simulink model "generic_truck"  (R2025a)
settings: Solver=VariableStepAuto  StartTime=0.0  StopTime=600  FixedStep=0.01  MaxStep=0.001  RelTol=1e-3  EnableMultiTasking=on
libraries: TruckMaker4SL x205, simulink x1
(part 6 of 9)

== matlab function generic_truck/TruckMaker/Two_TRack_Model/Two Track Model ==
  data: z input; u input; Q input; R input; xhat output; Ts input; P_out output; Fy_mean output; alpha_mean output; V_FL_whl output; V_FR_whl output; V_RL_whl output; V_RR_whl output
function [xhat,P_out,Fy_mean,alpha_mean,...
          V_FL_whl,V_FR_whl,V_RL_whl,V_RR_whl] ...
          = UKF_4Wheel(z,u,Q,R,Ts)

persistent x P

%% ================= INIT =================
if isempty(x)
    x = [15; 0; 0.01; 4; 4; 4; 4];
end

if isempty(P)
    P = diag([1 1 0.01 1e4 1e4 1e4 1e4]);
end

n = length(x);
m = length(z);

%% ================= VEHICLE =================
m_car = 7000;
Jz = 14232.357;
lf = 4.52;
lr = 0.95;
R_w = 0.49;
track=2.10;

%% ================= INPUTS =================
delta_FL = u(1);
delta_FR = u(2);
delta_RL = 0;
delta_RR = 0;

Fx_FL = u(5)/R_w;
Fx_FR = u(6)/R_w;
Fx_RL = u(7)/R_w;
Fx_RR = u(8)/R_w;

%% ================= ROTATION MATRICES =================
R_FL = [cos(delta_FL) sin(delta_FL);
       -sin(delta_FL) cos(delta_FL)];

R_FR = [cos(delta_FR) sin(delta_FR);
       -sin(delta_FR) cos(delta_FR)];

R_RL = eye(2);
R_RR = eye(2);

%% ================= GEOMETRY =================
tire_FL = [lf;  1.05; 0];
tire_FR = [lf; -1.05; 0];
tire_RL = [lr;  1.05; 0];
tire_RR = [lr; -1.05; 0];

CoM = [3.6; 0; 1];  % Ändra koor till COM (Jobba i CoG)  

rFL = tire_FL - CoM;
rFR = tire_FR - CoM;
rRL = tire_RL - CoM;
rRR = tire_RR - CoM;

%% ================= UKF =================
W0 = 1 - n/3;
Wi = (1 - W0)/(2*n);
gamma = sqrt(n/(1-W0));

%P = (P+P')/2 + 1e-9*eye(n); 
S = chol(P,'lower'); %% kolla upp den igen 

X = zeros(n,2*n+1);
X(:,1) = x;

for i=1:n
    X(:,i+1)   = x + gamma*S(:,i);
    X(:,i+1+n) = x - gamma*S(:,i);
end

%% ================= PROPAGATION =================
X_pred = zeros(n,2*n+1);
Fy_sigma = zeros(4,2*n+1);
alpha_sigma = zeros(4,2*n+1);
% R; M; Jz
for k=1:2*n+1

    vx = X(1,k);
    vy = X(2,k);
    r  = X(3,k);

    Cf_FL = X(4,k);
    Cf_FR = X(5,k);
    Cr_RL = X(6,k);
    Cr_RR = X(7,k);

    % ===== FIX 1: korrekt vx_safe =====
    %vx_safe = vx;

    Vc = [vx; vy; 0]; % vehilce Frame 
    omega = [0;0;r];

    V_FL = Vc + cross(omega,rFL);
    V_FR = Vc + cross(omega,rFR);
    V_RL = Vc + cross(omega,rRL);
    V_RR = Vc + cross(omega,rRR);

    V_FL_l = R_FL*V_FL(1:2);
    V_FR_l = R_FR*V_FR(1:2);
    V_RL_l = V_RL(1:2);
    V_RR_l = V_RR(1:2);
    
    %============Side Slip Vinkel på respektiv däck ==================
    alpha_FL = atan2(V_FL_l(2),max(abs(V_FL_l(1)),0.1));
    alpha_FR = atan2(V_FR_l(2),max(abs(V_FR_l(1)),0.1));
    alpha_RL = atan2(V_RL_l(2),max(abs(V_RL_l(1)),0.1));
    alpha_RR = atan2(V_RR_l(2),max(abs(V_RR_l(1)),0.1));


    %===================Forces==============================
    Fy_FL = -Cf_FL*alpha_FL;
    Fy_FR = -Cf_FR*alpha_FR;
    Fy_RL = -Cr_RL*alpha_RL;
    Fy_RR = -Cr_RR*alpha_RR;


    % Transformerta dessa krafter till kroppens FRAME
    F_FL = R_FL'*[Fx_FL;Fy_FL];
    F_FR = R_FR'*[Fx_FR;Fy_FR];
    F_RL = [Fx_RL;Fy_RL];
    F_RR = [Fx_RR;Fy_RR];

    Fx_sum = F_FL(1)+F_FR(1)+F_RL(1)+F_RR(1);
    Fy_sum = F_FL(2)+F_FR(2)+F_RL(2)+F_RR(2);

    dvx = Fx_sum/m_car + vy*r; % andra terma roteradnde koordinat system 
    dvy = Fy_sum/m_car - vx*r; 

%dW = truck.Jinv * (cross(R1, RotW1*F1) + cross(R2, RotW2*F2) 
                    % + cross(R3, F3) + cross(R4, F4));

    % ===== FIX 2: korrekt  eller ej fråga Axel  yaw moment =====
    % !!!!!!!!!!
    Mz = (lf-CoM(1))*(F_FL(2)+F_FR(2)) - (CoM(1)-lr)*(F_RL(2)+F_RR(2)) ... 
        + (track/2)*(F_FR(1)-F_FL(1)) + (track/2)*(F_RR(1)-F_RL(1));
    dr = Mz / Jz;

    X_pred(:,k) = [vx+dvx*Ts;
                   vy+dvy*Ts;
                   r+dr*Ts;
                   Cf_FL;
                   Cf_FR;
                   Cr_RL;
                   Cr_RR];

    Fy_sigma(:,k)    = [F_FL(2);F_FR(2);F_RL(2);F_RR(2)];
    alpha_sigma(:,k) = [alpha_FL;alpha_FR;alpha_RL;alpha_RR];
end

W = [W0 repmat(Wi,1,2*n)];
%x_pred = X_pred*W';
Fy_mean = Fy_sigma*W';
alpha_mean = alpha_sigma*W';
%% Predicted mean
x_pred = W0*X_pred(:,1);
for k=2:2*n+1
    x_pred = x_pred + Wi*X_pred(:,k);
end

%% ================= COVARIANCE =================
% P_pred = Q*Ts;
% for k=1:2*n+1
%     dx = X_pred(:,k)-x_pred;
%     P_pred = P_pred + W(k)*(dx*dx');
% end

%% Predicted covariance
P_pred = Q*Ts;
for k=1:2*n+1
    w = (k==1)*W0 + (k>1)*Wi;
    dx = X_pred(:,k) - x_pred;
    P_pred = P_pred + w*(dx*dx');
end
%% ================= MEASUREMENT =================
Z_sigma = zeros(m,2*n+1);

for k=1:2*n+1

    vx = X_pred(1,k);
    vy = X_pred(2,k);
    r  = X_pred(3,k);

    %Cf_FL = X_pred(4,k);
    %Cf_FR = X_pred(5,k);
    %Cr_RL = X_pred(6,k);
    %Cr_RR = X_pred(7,k);


    vx_safe = abs(vx);

    Vc = [vx_safe;vy;0];
    omega = [0;0;r];

    V_FL = Vc + cross(omega,rFL);
    V_FR = Vc + cross(omega,rFR);
    V_RL = Vc + cross(omega,rRL);
    V_RR = Vc + cross(omega,rRR);

    V_FL_l = R_FL*V_FL(1:2);
    V_FR_l = R_FR*V_FR(1:2);
    V_RL_l = V_RL(1:2);
    V_RR_l = V_RR(1:2);

     %============Side Slip Vinkel på respektiv däck ==================
    alpha_FL = atan2(V_FL_l(2),max(abs(V_FL_l(1)),0.1));
    alpha_FR = atan2(V_FR_l(2),max(abs(V_FR_l(1)),0.1));
    alpha_RL = atan2(V_RL_l(2),max(abs(V_RL_l(1)),0.1));
    alpha_RR = atan2(V_RR_l(2),max(abs(V_RR_l(1)),0.1));


    %===================Forces==============================
    Fy_FL = -Cf_FL*alpha_FL;
    Fy_FR = -Cf_FR*alpha_FR;
    Fy_RL = -Cr_RL*alpha_RL;
    Fy_RR = -Cr_RR*alpha_RR;


    % Transformerta dessa krafter till kroppens FRAME
    F_FL = R_FL'*[Fx_FL;Fy_FL];
    F_FR = R_FR'*[Fx_FR;Fy_FR];
    F_RL = [Fx_RL;Fy_RL];
    F_RR = [Fx_RR;Fy_RR];

    Fx_sum = F_FL(1)+F_FR(1)+F_RL(1)+F_RR(1);
    Fy_sum = F_FL(2)+F_FR(2)+F_RL(2)+F_RR(2);

    % ===== FIX 3: hjulhastigheter istället för krafter =====
    w_FL = V_FL_l(1)/R_w;    % Fråga MATS om Long slip och R_w 
    w_FR = V_FR_l(1)/R_w;
    w_RL = V_RL_l(1)/R_w;
    w_RR = V_RR_l(1)/R_w;

    ax = (Fx_sum)/m_car ;
    ay = (Fy_sum)/m_car;

    Z_sigma(:,k) = [ax; ay; vx; vy; r; w_FL; w_FR; w_RL; w_RR];
end

% z_pred = Z_sigma*W';
% 
% P_zz = R;
% P_xz = zeros(n,m);
% 
% for k=1:2*n+1
%     dz = Z_sigma(:,k)-z_pred;
%     dx = X_pred(:,k)-x_pred;
%     P_zz = P_zz + W(k)*(dz*dz');
%     P_xz = P_xz + W(k)*(dx*dz');
% end
% 
% %% ================= UPDATE =================
% K =   P_xz / P_zz;
% x = x_pred + K*(z - z_pred);
% 
% P = P_pred - K*P_zz*K';

% ===== FIX 4: symmetrisera P =====
%P = (P+P')/2 + 1e-9*eye(n);

%% Measurement mean
z_pred = W0*Z_sigma(:,1);
for k=2:2*n+1
    z_pred = z_pred + Wi*Z_sigma(:,k);
end

%% Measurement covariance
S_cov = R;
for k=1:2*n+1
    w = (k==1)*W0 + (k>1)*Wi;
    dz = Z_sigma(:,k) - z_pred;
    S_cov = S_cov + w*(dz*dz');
end

%% Cross covariance
Pxz = zeros(n,length(z));
for k=1:2*n+1
    w = (k==1)*W0 + (k>1)*Wi;
    dx = X_pred(:,k) - x_pred;
    dz = Z_sigma(:,k) - z_pred;
    Pxz = Pxz + w*(dx*dz');
end

%% Kalman update
K = Pxz / (S_cov);
x = x_pred + K*(z - z_pred);
P = P_pred - K*S_cov*K';

%% ================= OUTPUT =================
vx = x(1); vy = x(2); r = x(3);

Vc = [vx;vy;0];
omega = [0;0;r];

V_FL = Vc + cross(omega,rFL);
V_FR = Vc + cross(omega,rFR);
V_RL = Vc + cross(omega,rRL);
V_RR = Vc + cross(omega,rRR);

V_FL_whl = R_FL*V_FL(1:2);
V_FR_whl = R_FR*V_FR(1:2);
V_RL_whl = V_RL(1:2);
V_RR_whl = V_RR(1:2);

xhat =  x;
P_out = P;

end

== matlab function generic_truck/TruckMaker/Two_TRack_Model/Two Track Model1 ==
  data: z input; u input; Q input; R input; xhat output; Ts input; P_out output; Fy_mean output; alpha_mean output; V_FL_whl output; V_FR_whl output; V_RL_whl output; V_RR_whl output
function [xhat,P_out,Fy_mean,alpha_mean,...
          V_FL_whl,V_FR_whl,V_RL_whl,V_RR_whl] ...
          = UKF_4Wheel(z,u,Q,R,Ts)

persistent x P

%% ================= INIT =================
if isempty(x)
    x = [15; 0; 0.01; 10; 10; 10; 10];  % startvärden på cornering stiffness
end

if isempty(P)
    P = diag([1 1 0.01 1 1 1 1]);
end

n = length(x);
m = length(z);

%% ================= VEHICLE =================
m_car = 7000;
Jz = 14232.357;
lf = 4.52;
lr = 0.95;
R_w = 0.49;
track=2.10;
h_CoM = 1;  % höjd på CoM

%% ================= INPUTS =================
delta_FL = u(1);
delta_FR = u(2);
delta_RL = 0;
delta_RR = 0;

Fx_FL = u(5)/R_w;
Fx_FR = u(6)/R_w;
Fx_RL = u(7)/R_w;
Fx_RR = u(8)/R_w;

%% ================= ROTATION MATRICES =================
R_FL = [cos(delta_FL) sin(delta_FL);
       -sin(delta_FL) cos(delta_FL)];

R_FR = [cos(delta_FR) sin(delta_FR);
       -sin(delta_FR) cos(delta_FR)];

R_RL = eye(2);
R_RR = eye(2);

%% ================= GEOMETRY =================
tire_FL = [lf;  track/2; 0];
tire_FR = [lf; -track/2; 0];
tire_RL = [lr;  track/2; 0];
tire_RR = [lr; -track/2; 0];

CoM = [3.6; 0; h_CoM];  

rFL = tire_FL - CoM;
rFR = tire_FR - CoM;
rRL = tire_RL - CoM;
rRR = tire_RR - CoM;

%% ================= UKF =================
W0 = 1 - n/3;
Wi = (1 - W0)/(2*n);
gamma = sqrt(n/(1-W0));

S = chol(P,'lower');

X = zeros(n,2*n+1);
X(:,1) = x;

for i=1:n
    X(:,i+1)   = x + gamma*S(:,i);
    X(:,i+1+n) = x - gamma*S(:,i);
end

%% ================= PROPAGATION =================
X_pred = zeros(n,2*n+1);
Fy_sigma = zeros(4,2*n+1);
alpha_sigma = zeros(4,2*n+1);

for k=1:2*n+1

    vx = X(1,k);
    vy = X(2,k);
    r  = X(3,k);

    Cf_FL = X(4,k);
    Cf_FR = X(5,k);
    Cr_RL = X(6,k);
    Cr_RR = X(7,k);

    Vc = [vx; vy; 0];
    omega = [0;0;r];

    V_FL = Vc + cross(omega,rFL);
    V_FR = Vc + cross(omega,rFR);
    V_RL = Vc + cross(omega,rRL);
    V_RR = Vc + cross(omega,rRR);

    V_FL_l = R_FL*V_FL(1:2);
    V_FR_l = R_FR*V_FR(1:2);
    V_RL_l = V_RL(1:2);
    V_RR_l = V_RR(1:2);
    
    % Side slip angles
    alpha_FL = atan2(V_FL_l(2),max(abs(V_FL_l(1)),0.1));
    alpha_FR = atan2(V_FR_l(2),max(abs(V_FR_l(1)),0.1));
    alpha_RL = atan2(V_RL_l(2),max(abs(V_RL_l(1)),0.1));
    alpha_RR = atan2(V_RR_l(2),max(abs(V_RR_l(1)),0.1));

    % ================= LOAD TRANSFER =================
    Fz_FL = m_car/4*9.81 - m_car*r*vy - m_car*vx^2*lr/(lf+lr); % enkel approx
    Fz_FR = m_car/4*9.81 - m_car*r*vy - m_car*vx^2*lr/(lf+lr);
    Fz_RL = m_car/4*9.81 + m_car*r*vy + m_car*vx^2*lf/(lf+lr);
    Fz_RR = m_car/4*9.81 + m_car*r*vy + m_car*vx^2*lf/(lf+lr);

    % ================= FORCES =================
    Fy_FL = -Cf_FL * Fz_FL * alpha_FL;
    Fy_FR = -Cf_FR * Fz_FR * alpha_FR;
    Fy_RL = -Cr_RL * Fz_RL * alpha_RL;
    Fy_RR = -Cr_RR * Fz_RR * alpha_RR;

    F_FL = R_FL'*[Fx_FL;Fy_FL];
    F_FR = R_FR'*[Fx_FR;Fy_FR];
    F_RL = [Fx_RL;Fy_RL];
    F_RR = [Fx_RR;Fy_RR];

    Fx_sum = F_FL(1)+F_FR(1)+F_RL(1)+F_RR(1);
    Fy_sum = F_FL(2)+F_FR(2)+F_RL(2)+F_RR(2);

    dvx = Fx_sum/m_car + vy*r;
    dvy = Fy_sum/m_car - vx*r;

    Mz = (lf-CoM(1))*(F_FL(2)+F_FR(2)) - (CoM(1)-lr)*(F_RL(2)+F_RR(2)) ...
        + (track/2)*(F_FR(1)-F_FL(1)) + (track/2)*(F_RR(1)-F_RL(1));
    dr = Mz / Jz;

    X_pred(:,k) = [vx+dvx*Ts;
                   vy+dvy*Ts;
                   r+dr*Ts;
                   Cf_FL;
                   Cf_FR;
                   Cr_RL;
                   Cr_RR];

    Fy_sigma(:,k)    = [F_FL(2);F_FR(2);F_RL(2);F_RR(2)];
    alpha_sigma(:,k) = [alpha_FL;alpha_FR;alpha_RL;alpha_RR];
end

%% ================= UKF MEAN & COVARIANCE =================
W = [W0 repmat(Wi,1,2*n)];
Fy_mean = Fy_sigma*W';
alpha_mean = alpha_sigma*W';

% State mean
x_pred = W0*X_pred(:,1);
for k=2:2*n+1
    x_pred = x_pred + Wi*X_pred(:,k);
end

% State covariance
P_pred = Q*Ts;
for k=1:2*n+1
    w = (k==1)*W0 + (k>1)*Wi;
    dx = X_pred(:,k) - x_pred;
    P_pred = P_pred + w*(dx*dx');
end

%% ================= MEASUREMENT =================
Z_sigma = zeros(m,2*n+1);

for k=1:2*n+1
    vx = X_pred(1,k);
    vy = X_pred(2,k);
    r  = X_pred(3,k);

    Cf_FL = X_pred(4,k);
    Cf_FR = X_pred(5,k);
    Cr_RL = X_pred(6,k);
    Cr_RR = X_pred(7,k);

    Vc = [vx;vy;0];
    omega = [0;0;r];

    V_FL = Vc + cross(omega,rFL);
    V_FR = Vc + cross(omega,rFR);
    V_RL = Vc + cross(omega,rRL);
    V_RR = Vc + cross(omega,rRR);

    V_FL_l = R_FL*V_FL(1:2);
    V_FR_l = R_FR*V_FR(1:2);
    V_RL_l = V_RL(1:2);
    V_RR_l = V_RR(1:2);

    alpha_FL = atan2(V_FL_l(2),max(abs(V_FL_l(1)),0.1));
    alpha_FR = atan2(V_FR_l(2),max(abs(V_FR_l(1)),0.1));
    alpha_RL = atan2(V_RL_l(2),max(abs(V_RL_l(1)),0.1));
    alpha_RR = atan2(V_RR_l(2),max(abs(V_RR_l(1)),0.1));

     % ================= LOAD TRANSFER =================
    Fz_FL = m_car/4*9.81 - m_car*r*vy - m_car*vx^2*lr/(lf+lr); % enkel approx
    Fz_FR = m_car/4*9.81 - m_car*r*vy - m_car*vx^2*lr/(lf+lr);
    Fz_RL = m_car/4*9.81 + m_car*r*vy + m_car*vx^2*lf/(lf+lr);
    Fz_RR = m_car/4*9.81 + m_car*r*vy + m_car*vx^2*lf/(lf+lr);

    Fy_FL = -Cf_FL * Fz_FL * alpha_FL;
    Fy_FR = -Cf_FR * Fz_FR * alpha_FR;
    Fy_RL = -Cr_RL * Fz_RL * alpha_RL;
    Fy_RR = -Cr_RR * Fz_RR * alpha_RR;

    F_FL = R_FL'*[Fx_FL;Fy_FL];
    F_FR = R_FR'*[Fx_FR;Fy_FR];
    F_RL = [Fx_RL;Fy_RL];
    F_RR = [Fx_RR;Fy_RR];

    Fx_sum = F_FL(1)+F_FR(1)+F_RL(1)+F_RR(1);
    Fy_sum = F_FL(2)+F_FR(2)+F_RL(2)+F_RR(2);

    w_FL = V_FL_l(1)/R_w;
    w_FR = V_FR_l(1)/R_w;
    w_RL = V_RL_l(1)/R_w;
    w_RR = V_RR_l(1)/R_w;

    ax = Fx_sum/m_car;
    ay = Fy_sum/m_car;

    Z_sigma(:,k) = [ax; ay; vx; vy; r; w_FL; w_FR; w_RL; w_RR];
end

%% ================= UKF UPDATE =================
% Measurement mean
z_pred = W0*Z_sigma(:,1);
for k=2:2*n+1
    z_pred = z_pred + Wi*Z_sigma(:,k);
end

% Measurement covariance
S_cov = R;
for k=1:2*n+1
    w = (k==1)*W0 + (k>1)*Wi;
    dz = Z_sigma(:,k) - z_pred;
    S_cov = S_cov + w*(dz*dz');
end

% Cross covariance
Pxz = zeros(n,length(z));
for k=1:2*n+1
    w = (k==1)*W0 + (k>1)*Wi;
    dx = X_pred(:,k) - x_pred;
    dz = Z_sigma(:,k) - z_pred;
    Pxz = Pxz + w*(dx*dz');
end

% Kalman update
K = Pxz / S_cov;
x = x_pred + K*(z - z_pred);
P = P_pred - K*S_cov*K';

%% ================= OUTPUT =================
vx = x(1); vy = x(2); r = x(3);

Vc = [vx;vy;0];
omega = [0;0;r];

V_FL = Vc + cross(omega,rFL);
V_FR = Vc + cross(omega,rFR);
V_RL = Vc + cross(omega,rRL);
V_RR = Vc + cross(omega,rRR);

V_FL_whl = R_FL*V_FL(1:2);
V_FR_whl = R_FR*V_FR(1:2);
V_RL_whl = V_RL(1:2);
V_RR_whl = V_RR(1:2);

xhat =  x;
P_out = P;
Fy_mean = Fy_mean;
alpha_mean = alpha_mean;

end

== matlab function generic_truck/TruckMaker/Subsystem1/ONE_TRACK_MODEL_TRACTOR_UKF/MATLAB Function ==
  data: z input; u input; Cf output; Cr output; alpha_f output; alpha_r output
function [Cf, Cr, alpha_f, alpha_r] = stiffness_computation(z, u)
%
% Signal: z = [ ax; ay; az; 
%               vx; vy; vz;
%               rx; ry; rz;
%               alphax; alphay; alphaz;
%               wFL; wFR; wRL; wRR; ]
%
%         u = [ delta; T_rl; T_rr; ]
%

% ------------------------------------------------------------------------%
% Physics
% ------------------------------------------------------------------------%

g = 9.82; % [m/s^2]

% ------------------------------------------------------------------------%
% Truck Parameters
% ------------------------------------------------------------------------%

% Mass [kg]
m = 6800;

% Inertial tensor [kg m^2]
J = [
     5430.025, 0.000,    -589.488;
     0.000,    9407.562,  0.000;
    -589.488,  0.000,     12994.917;
];

% Position vectors [m]
p_cog  = [3.473, 0.000, 0.925].';  % Center of Gravity
p_fax  = [4.520, 0.000, 0.490].';  % Front axle
p_rax  = [0.950, 0.000, 0.490].';  % Rear axle
p_bod  = [3.600, 0.000, 1.000].';  % Body frame
p_imu  = p_bod;

% p_wfl  = [4.520,  1.050, 0.490].'; % Front wheel left
% p_wfr  = [4.520, -1.050, 0.490].'; % Front wheel right
% 
% p_wrl  = [0.950,  1.050, 0.490].'; % Rear wheel left
% p_wrcl = [0.950,  0.860, 0.490].'; % Rear wheel carrier left
% p_wrcr = [0.950, -0.860, 0.490].'; % Rear wheel carrier right
% p_wrr  = [0.950, -1.050, 0.490].'; % Rear wheel right
% 
% Axle load
% m_f = 4805.882; % [kg]
% m_r = 2194.118; % [kg]
% 
% Wheel base
% long = [1,0,0] * abs(p_fax - p_rax); % length [m]
% wide = [0,1,0] * abs(p_wrr - p_wrl); % width  [m]

% CoG hight
high = p_cog(3);

% Wheel radius
% Rwf = 0.505;
% Rwr = 0.505;

% longitudinal distance from cog to axles
lf = [1,0,0] * abs(p_fax - p_cog);
lr = [1,0,0] * abs(p_rax - p_cog);

% ------------------------------------------------------------------------%
% Inputs
% ------------------------------------------------------------------------%

a =  [z(1:2);0]; % IMU acceleration
v =  [z(3:4);0]; % IMU velocity

alpha = [0;0;0];     % IMU yaw acceleration

omega = [0;0;z(end)];  % IMU yaw rate


delta = u(1); % steering angle of one-track front wheel (pre-computed)

T_rl = u(2); % rear left  torque (not used)
T_rr = u(3); % rear right torque (not used)
 
% ------------------------------------------------------------------------%
% Translate measurements
% ------------------------------------------------------------------------%

% displacement vectors
Rfax = p_fax - p_imu; Rfax(3) = -p_imu(3); % straight projection to contact
Rrax = p_rax - p_imu; Rrax(3) = -p_imu(3); % --||--
Rcog = p_cog - p_imu;

% rotation matrix
Rotf = [ 
   cos(delta), -sin(delta), 0;
   sin(delta),  cos(delta), 0;
            0,           0, 1;
];

% velocity translation
% --------------------
vf = Rotf.' * (v + cross(omega, Rfax));
vr = eye(3) * (v + cross(omega, Rrax));

% acceleration translation 
% ------------------------
acog = a + cross(omega, cross(omega, Rcog)) + cross(alpha, Rcog);

% ------------------------------------------------------------------------%
% Computation
% ------------------------------------------------------------------------%

% lateral forces
% --------------
%Ffy = (J(3,3)*alpha(3)+m*acog(2)*lr) / (long * cos(delta));
%Fry = (m*acog(2)*lf - J(3,3)*alpha(3)) / long;

Ffy = (acog(2)*lr) / cos(delta);
Fry = (acog(2)*lf);

% slip
% ----
alpha_f = atan2(vf(2), max(abs(vf(1)), .1));
alpha_r = atan2(vr(2), max(abs(vr(1)), .1));

% normal forces
% -------------
%Ffz = m*g*lr/long - m*acog(1)*high/long;
%Frz = m*g*lf/long + m*acog(1)*high/long;

Ffz = g*lr - acog(1)*high;
Frz = g*lf + acog(1)*high;

% normalized coefficients
% -----------------------
Cf = Ffy / (alpha_f * Ffz); % reference 
Cr = Fry / (alpha_r * Frz); % reference

== matlab function generic_truck/TruckMaker/Subsystem1/ONE_TRACK_MODEL_TRACTOR_UKF/UKF_ONE_TRACK1 ==
  data: z input; u input; xhat output; Q input; R input; Ts input; P output; dxdt output; innovation output; K_out output; S_out output; z_pred_out output; data input
function [xhat, P, dxdt, innovation, K_out, S_out, z_pred_out] = UKF_TruckTrailer(z,u,Q,R,Ts,data)
persistent x Pk dxdt_old t

%% =========================
%% INIT
%% =========================
if isempty(x)
    x = [15;0.1;0.1;7.5;7.5;0;0;6]; % [vx vy wz Cf Cr psi wz_tr Cr_tr]
end
if isempty(Pk)
    Pk = diag([0.1 0.1 0.1 5 5 0.1 0.1 5]);
end
if isempty(dxdt_old)
    dxdt_old = zeros(8,1);
end
if isempty(t)
    t = 0;
end

t = data;
if t < 30
    xhat=x; P=Pk; dxdt=dxdt_old;
    
    innovation=zeros(length(z),1);
    K_out=zeros(length(x), length(z));
    S_out=eye(length(z));
    z_pred_out=zeros(length(z),1);
    return
end

%% =========================
%% CONSTANTS
%% =========================
g = 9.82;
% Truck
m = 6800; Jz = 12994.917; Rwheel = 0.49;
w_track = 2.1; % FIXED: Lade till spårvidd för att kunna differentiera hjulhastigheter
% Trailer
m_tr = 31960; Jz_tr = 145971.764;

% Geometry &  koordinat punkter på Truck
p_cog = [3.473;0;0.925];
p_fax = [4.520;0;0.490];
p_rax = [0.950;0;0.490];
p_imu = [3.600;0;1.000];
hitch = [1.9;0;1.21];
Rcog = p_imu - p_cog;

% Geometry Trailer
p_cog_tr = [-6.195;0;1.95];
p_rax_tr = [-9.0;0;0.490];
hitch_tr = [-1.25;0;1.25];

lf = abs(p_fax(1)-p_cog(1)); 
lr = abs(p_cog(1)-p_rax(1)); 
L = lf + lr;
h = p_cog(3);

Rfax = p_fax - p_cog; Rfax(3)=-p_cog(3);
Rrax = p_rax - p_cog; Rrax(3)=-p_cog(3);
Rhitch = hitch - p_cog;
lhitch = Rhitch(1);

lfhitch = abs(p_fax(1) -hitch(1));

lf_tr = abs(hitch_tr(1)-p_cog_tr(1));

lr_tr = abs(p_cog_tr(1)-p_rax_tr(1));

L_tr = lf_tr + lr_tr;
h_tr = p_cog_tr(3);
hHitch= hitch(3);

Rrax_tr = p_rax_tr - hitch_tr; Rrax_tr(3)=-hitch_tr(3);

%% =========================
%% INPUTS
%% =========================
delta = u(1); % steering to road angle 

% Rear wheel drive
T_rl = u(2);   
T_rr = u(3);

Fxh = u(4); % kraft på dragkrok uttryckt i släpets koordinatsystem
Fyh = u(5); 

Fx_vehicle = (T_rl+T_rr)/Rwheel;

%% =========================
%% UKF PARAMS
%% =========================
n = length(x);
nSPx = 2*n+1;
W0 = 1 - n/3;
Wi = (1 - W0)/(2*n);
gamma = sqrt(n/(1 - W0));

%% =========================
%% SIGMA POINTS (PRIOR)
%% =========================
Pk = (Pk+Pk')/2 + 1e-9*eye(n);
Sx = chol(Pk,'lower');
X_pre = zeros(n,nSPx);
X_pre(:,1) = x;
for i=1:n
    X_pre(:,i+1)   = x + gamma*Sx(:,i);
    X_pre(:,i+1+n) = x - gamma*Sx(:,i);
end

%% =========================
%% PREDICTION
%% =========================
X_pred = zeros(n,nSPx);
dxdt_model = zeros(n,1);
for k=1:nSPx
    Xk = X_pre(:,k);
    
    % Traktor CoG
    vx=Xk(1); vy=Xk(2); wz=Xk(3);
    Cf=Xk(4); Cr=Xk(5);
    
    % Trailer 
    psi=Xk(6); wz_tr=Xk(7); Cr_tr=Xk(8);
    
    v_cog=[vx;vy;0];
    omega=[0;0;wz];
    
    %% ===== TRAILER =====
    v_hitch_truck = v_cog + cross(omega,Rhitch);
    Rot_tr=[cos(psi) -sin(psi) 0;
            sin(psi)  cos(psi) 0;
            0 0 1];
    omega_tr=[0;0;wz_tr];
    
    % FIXED: Tog bort minustecknet framför Rot_tr för konsekvens
    v_hitch_trailer = Rot_tr.' * v_hitch_truck; 
    
    % velocity of trailer wheel at rear axle contact point  
    v_tr_ax = v_hitch_trailer + cross(omega_tr,Rrax_tr);
    
    % slip
    alpha_tr = atan2(v_tr_ax(2),max(abs(v_tr_ax(1)),0.1));
    
    % load transfer approximation 
    ax_tr = Fxh/m_tr;
    
    % FIXED: Ändrade till minustecken eftersom acceleration flyttar vikten bakåt från dragkroken
    Fz_hitch = m_tr*g*lr_tr/L_tr - m_tr*ax_tr*(h_tr-hHitch)/L_tr;
    Fz_tr    = m_tr*g - Fz_hitch;
    
    % Brush Model 
    Fy_tr = -Cr_tr*alpha_tr*Fz_tr;
    
    %% ===== TRUCK =====
    % Rotation Matris 
    Rotf=[cos(delta) -sin(delta) 0;
          sin(delta)  cos(delta) 0;
          0                0     1];
    
    % velocities at contact point 
    vf = Rotf.'*(v_cog + cross(omega,Rfax));
    vr = v_cog + cross(omega,Rrax);
    
    % slip per wheel 
    alpha_f = atan2(vf(2),max(abs(vf(1)),0.1));
    alpha_r = atan2(vr(2),max(abs(vr(1)),0.1));
    
    F_hitch_trailer=[u(4);u(5);0];
    F_hitch_body= Rot_tr.' * F_hitch_trailer;
    
    % load transfer approximation
    ax_est = (Fx_vehicle - F_hitch_body(1))/m; % Använder förenklad acceleration utan coriolis för lastöverföring
    
    % FIXED: Exakt momentbalans för Ffz och Frz. Tar hänsyn till var dragkroken faktiskt sitter.
    Ffz = (m*g*lr - m*ax_est*h + Fz_hitch*(hitch(1) - p_rax(1)) - F_hitch_body(1)*hHitch) / L;
    Frz = (m*g*lf + m*ax_est*h + Fz_hitch*(p_fax(1) - hitch(1)) + F_hitch_body(1)*hHitch) / L;
    
    % Säkerhetsspärr mot negativ normalkraft i extrema transienter
    %Ffz = max(Ffz, 100);
    %Frz = max(Frz, 100);

    % brush model 
    Fy_f = -Cf*alpha_f*Ffz;
    Fy_r = -Cr*alpha_r*Frz;
    
    %% ===== DYNAMICS =====
    dvx = (Fx_vehicle - Fy_f*sin(delta) - F_hitch_body(1))/m + vy*wz;
    dvy = (Fy_f*cos(delta) + Fy_r - F_hitch_body(2))/m - vx*wz;
    
    % FIXED: Återinförde dragkrokens sidokraft i lastbilens gir-ekvation
    dwz = (lf*Fy_f*cos(delta) - lr*Fy_r - lhitch*(F_hitch_body(2)))/Jz;
    
    dpsi = wz_tr - wz; % Articulation angle 
    dwz_tr = (lr_tr*Fy_tr - lf_tr*Fyh)/Jz_tr;
    
    if k==1
        dxdt_model=[dvx;dvy;dwz;0;0;dpsi;dwz_tr;0];
    end
    
    X_pred(:,k) = Xk + Ts*[dvx;
                           dvy;
                           dwz;
                           0;
                           0;
                           dpsi;
                           dwz_tr;
                           0];
end

%% ===== MEAN & COV
x_pred=zeros(n,1);
P_pred=zeros(n);
for k=1:nSPx
    w=(k==1)*W0+(k>1)*Wi;
    x_pred=x_pred+w*X_pred(:,k);
end
for k=1:nSPx
    w=(k==1)*W0+(k>1)*Wi;
    dx=X_pred(:,k)-x_pred;
    P_pred=P_pred+w*(dx*dx');
end
P_pred=P_pred+Q*Ts;
P_pred=(P_pred+P_pred')/2 + 1e-9*eye(n);

%% =========================
%% MEASUREMENT
%% =========================
Sx=chol(P_pred,'lower');
X_post=zeros(n,nSPx);
X_post(:,1)=x_pred;
for i=1:n
    X_post(:,i+1)  =x_pred + gamma*Sx(:,i);
    X_post(:,i+1+n)=x_pred - gamma*Sx(:,i);
end

Z=zeros(length(z),nSPx);
for k=1:nSPx
    Xk=X_post(:,k);
    
    % Traktor CoG
    vx=Xk(1); vy=Xk(2); wz=Xk(3);
    Cf=Xk(4); Cr=Xk(5);
    
    % Trailer 
    psi=Xk(6); wz_tr=Xk(7); Cr_tr=Xk(8); 
    
    v_cog=[vx;vy;0];
    omega=[0;0;wz];
    
    %% ===== TRAILER =====
    v_hitch_truck = v_cog + cross(omega,Rhitch);
    Rot_tr=[cos(psi) -sin(psi) 0;
            sin(psi)  cos(psi) 0;
            0 0 1];
    omega_tr=[0;0;wz_tr];
    
    v_hitch_trailer = Rot_tr.' * v_hitch_truck;
    
    v_tr_ax = v_hitch_trailer + cross(omega_tr,Rrax_tr);
    alpha_tr = atan2(v_tr_ax(2),max(abs(v_tr_ax(1)),0.1));
    
    ax_tr = Fxh / m_tr; 
    
    % FIXED: Ändrade till minustecken
    Fz_hitch = m_tr*g*lr_tr/L_tr - m_tr*ax_tr*(h_tr-hHitch)/L_tr;
    Fz_tr = m_tr*g - Fz_hitch;
    
    Fy_tr = -Cr_tr*alpha_tr*Fz_tr;
    
    %% ===== TRUCK =====    
    Rotf=[cos(delta) -sin(delta) 0;
          sin(delta)  cos(delta) 0;
          0                0     1];
    
    vf = Rotf.'*(v_cog + cross(omega,Rfax));
    vr = v_cog + cross(omega,Rrax);
    
    alpha_f = atan2(vf(2),max(abs(vf(1)),0.1));
    alpha_r = atan2(vr(2),max(abs(vr(1)),0.1));
    
    F_hitch_trailer=[u(4);u(5);0];
    F_hitch_body= Rot_tr.'* F_hitch_trailer;
    
    ax_est = (Fx_vehicle - F_hitch_body(1))/m;
    
    % FIXED: Samma exakta momentbalans som i prediktionsloopen
    Ffz = (m*g*lr - m*ax_est*h + Fz_hitch*(hitch(1) - p_rax(1)) - F_hitch_body(1)*hHitch) / L;
    Frz = (m*g*lf + m*ax_est*h + Fz_hitch*(p_fax(1) - hitch(1)) + F_hitch_body(1)*hHitch) / L;
    
    %Ffz = max(Ffz, 100);
    %Frz = max(Frz, 100);
    
    Fy_f = -Cf*alpha_f*Ffz;
    Fy_r = -Cr*alpha_r*Frz;
    
    %% ===== DYNAMICS (for sensors) =====
    % FIXED: Döpte om dessa till a_specific_x/y för att inte blanda ihop med tillståndsderivatan
    % En IMU mäter inte coriolis, därav ingen vy*wz term här
    a_specific_x = (Fx_vehicle - Fy_f*sin(delta) - F_hitch_body(1))/m;
    a_specific_y = (Fy_f*cos(delta) + Fy_r - F_hitch_body(2))/m;
    
    % Återinförde släpets moment
    dwz = (lf*Fy_f*cos(delta) - lr*Fy_r - lhitch*(F_hitch_body(2)))/Jz;
    
    a_cog = [a_specific_x; a_specific_y; 0];
    alpha_vec = [0; 0; dwz];
    
    a_imu = a_cog + cross(omega,cross(omega,Rcog)) + cross(alpha_vec,Rcog);
    v_imu = v_cog + cross(omega,Rcog);
    
    % FIXED: Lade till spårvidd för att få korrekta differenser vid svängning
    omega_rl = (vx - wz * w_track/2) / Rwheel;
    omega_rr = (vx + wz * w_track/2) / Rwheel;
    omega_tr_ML = (v_tr_ax(1) - wz_tr * w_track/2) / Rwheel;
    omega_tr_MR = (v_tr_ax(1) + wz_tr * w_track/2) / Rwheel;
    
    Z(:,k)=[a_imu(1:2); v_imu(1); v_imu(2); wz; omega_rl; omega_rr; omega_tr_ML; omega_tr_MR];
end

%% ===== REST (sensor selection + update) =====
z_pred=zeros(length(z),1);
for k=1:nSPx
    w=(k==1)*W0+(k>1)*Wi;
    z_pred=z_pred+w*Z(:,k);
end

valid_idx=true(length(z),1);
valid_idx=valid_idx & ~isnan(z);
z_used=z(valid_idx);
z_pred_used=z_pred(valid_idx);
Z_used=Z(valid_idx,:);
R_used=R(valid_idx,valid_idx);

S_cov=zeros(length(z_used));
Pxz=zeros(n,length(z_used));
for k=1:nSPx
    w=(k==1)*W0+(k>1)*Wi;
    dz=Z_used(:,k)-z_pred_used;
    dx=X_post(:,k)-x_pred;
    S_cov=S_cov+w*(dz*dz');
    Pxz=Pxz+w*(dx*dz');
end

S_cov=S_cov+R_used;
S_cov=(S_cov+S_cov')/2 + 1e-9*eye(size(S_cov));
K=Pxz/S_cov;

x=x_pred + K*(z_used - z_pred_used);
Pk=P_pred - K*S_cov*K';
Pk=(Pk+Pk')/2 + 1e-9*eye(n);

%% OUTPUT
xhat=x;
P=Pk;
dxdt=dxdt_model;

innovation=zeros(length(z),1);
innovation(valid_idx)=z_used - z_pred_used;
K_out=zeros(n,length(z));
K_out(:,valid_idx)=K;
S_out=zeros(length(z));
S_out(valid_idx,valid_idx)=S_cov;
z_pred_out=z_pred;

end

== matlab function generic_truck/TruckMaker/Subsystem1/EKF_ONE_TRACK ==
  data: z input; u input; xhat output; Q input; R input; Ts input; P output
function [xhat, P] = EKF_Bicycle_Full_NoBias(z, u, Q, R, Ts)
% EKF for One-Track / Bicycle Model (No IMU Bias)
% States: x = [vx; vy; r; Cf; Cr]
% Measurements: z = [ax; ay; vx; vy; r; wL; wR]

%% ---------------- Persistent safe initialization ----------------
persistent x Pk initialized

% Säker initialisering
if isempty(x)
    x = [15; 0; 0.05; 2e4; 2e4];  % vx, vy, r, Cf, Cr
end

if isempty(Pk)
    Pk = diag([1 1 0.05 4e4 4e4].^2); % 5x5
end

if isempty(initialized)
    initialized = true;
end


%% ---------------- Vehicle parameters ----------------

m  = 6800;        %  mass
g  = 9.82;        % gravity contanst   
Jz = 12994.917;   % yaw interia
Rw = 0.49;          % wheel radius
width = 2.49;       % track width

p_cog  = [3.473; 0; 0.925];
p_fax  = [4.520; 0; 0.490];

p_rax  = [0.950; 0; 0.490];
p_imu  = [3.600; 0; 1.000];

lf = abs(p_fax(1)-p_cog(1));   % front CoG distance
lr = abs(p_cog(1)-p_rax(1));   % rear CoG distance
L  = lf + lr;
h  = p_cog(3);

Rfax = p_fax - p_imu; Rfax(3) = -p_imu(3);
Rrax = p_rax - p_imu; Rrax(3) = -p_imu(3);
Rcog = p_cog - p_imu;

%% ---------------- Inputs ----------------
delta = u(1);                             % Average steering Angle (FL +FR)/2
T_rl  = u(2);                             % torque RL  
T_rr  = u(3);                             %torque RR
Rwheel = 0.49;                            % wheel radius
Fx_vehicle = (T_rl + T_rr)/Rwheel;        % longitudinal force

%% ---------------- States ----------------
vx = x(1); vy = x(2); r = x(3); Cf = x(4); Cr= x(5);

Rotf = [ cos(delta)     -sin(delta)     0;
         sin(delta)      cos(delta)     0;
             0              0           1];

v_cog = [vx; vy; 0];
omega = [0;0;r];

% Contact patch velocities
vf = Rotf.' * (v_cog + cross(omega,Rfax));
vr = v_cog + cross(omega,Rrax);

alpha_f = atan2(vf(2), max(abs(vf(1)),0.1));
alpha_r = atan2(vr(2), max(abs(vr(1)),0.1));

% Longitudinal accel estimate to compute the vertikel forces
dvx_temp = Fx_vehicle/m + vy*r;

% Normal forces
Ffz = m*g*lr/L - m*dvx_temp*h/L;
Frz = m*g*lf/L + m*dvx_temp*h/L;

% Tire forces
Fy_f = Cf * alpha_f * Ffz;
Fy_r = Cr * alpha_r * Frz;

% Full dynamics 
dvx = (Fx_vehicle - Fy_f*sin(delta))/m + vy*r;
dvy = (Fy_f*cos(delta) + Fy_r)/m - vx*r;
dr  = (lf*Fy_f*cos(delta) - lr*Fy_r)/Jz;

% State propagation
xdot = [dvx; dvy; dr; 0; 0];
x_pred = x + Ts*xdot;

%% ---------------- Jacobian F ----------------
F= zeros(5,5);
F(1,:) = [                                1 - (Cf*Ts*sin(delta)*(vy + lf*r))/(m*vx^2),              Ts*(r + (Cf*sin(delta))/(m*vx)),                   Ts*(vy + (Cf*lf*sin(delta))/(m*vx)),    -(Ts*sin(delta)*(delta - (vy + lf*r)/vx))/m,                            0];
F(2,:) = [  -Ts*(r - ((Cr*(vy - lr*r))/vx^2 + (Cf*cos(delta)*(vy + lf*r))/vx^2)/m),      1 - (Ts*(Cr/vx + (Cf*cos(delta))/vx))/m,    -Ts*(vx - ((Cr*lr)/vx - (Cf*lf*cos(delta))/vx)/m),     (Ts*cos(delta)*(delta - (vy + lf*r)/vx))/m,    -(Ts*(vy - lr*r))/(m*vx)];
F(3,:) = [-(Ts*((Cr*lr*(vy - lr*r))/vx^2 - (Cf*lf*cos(delta)*(vy + lf*r))/vx^2))/Jz, (Ts*((Cr*lr)/vx - (Cf*lf*cos(delta))/vx))/Jz, 1 - (Ts*((Cf*cos(delta)*lf^2)/vx + (Cr*lr^2)/vx))/Jz, (Ts*lf*cos(delta)*(delta - (vy + lf*r)/vx))/Jz, (Ts*lr*(vy - lr*r))/(Jz*vx)];
F(4,:) = [                                                                            0,                                              0,                                                      0,                                                 1,                            0];
F(5,:) = [                                                                            0,                                              0,                                                      0,                                                 0,                            1];


%% ---------------- Covariance prediction ----------------
P_pred = F*Pk*F' + Q;

%% ---------------- Measurement model ----------------
ax_hat = dvx -  vy*r;                % longitudinal accel
ay_hat = dvy + vx*r;                % lateral accel
%vx_hat = vx;
%vy_hat = vy;
%r_hat  = r;
%wL_hat = (vx - width/2 * r)/Rw;
%wR_hat = (vx + width/2 * r)/Rw;

a_cog = [ax_hat; ay_hat; 0];
alpha_vec = [0;0;dr];

% Transform to IMU
a_imu = a_cog - cross(omega, cross(omega,Rcog))- cross(alpha_vec,Rcog);
v_imu = v_cog + cross(omega,Rcog);

z_hat = [a_imu(1:2);
         v_imu(1:2);
         alpha_vec(3);
         omega(3)];

%z_hat = [ax_hat; ay_hat; vx_hat; vy_hat; dr_hat r_hat; wL_hat; wR_hat];

%% ---------------- Measurement Jacobian H ----------------
H = zeros(size(z_hat,1),size(x,1));

%H = zeros(7,5);
H(1,:) = [                               1 - (Cf*Ts*sin(delta)*(vy + lf*r))/(m*vx^2),         Ts*(r + (Cf*sin(delta))/(m*vx)) - r,                      Ts*(vy + (Cf*lf*sin(delta))/(m*vx)) - vy, -(Ts*sin(delta)*(delta - (vy + lf*r)/vx))/m,                            0];
H(2,:) = [-Ts*(r - ((Cr*(vy - lr*r))/vx^2 + (Cf*cos(delta)*(vy + lf*r))/vx^2)/m), 1 - (Ts*(Cr/vx + (Cf*cos(delta))/vx))/m, vx - Ts*(vx - ((Cr*lr)/vx - (Cf*lf*cos(delta))/vx)/m),  (Ts*cos(delta)*(delta - (vy + lf*r)/vx))/m, -(Ts*(vy - lr*r))/(m*vx)];
H(3,:) = [                                                                             1,                                               0,                                                                 0,                                               0,            0];
H(4,:) = [                                                                             0,                                               1,                                                                 0,                                               0,            0];
H(5,:) = [                                                                             0,                                               0,                                                                 0,                                               0,            0];
H(6,:) = [                                                                             0,                                               0,                                                                 1,                                               0,            0];
%H(7,:) = [                                                                             1/Rw,                                            0,                                                     -width/(2*Rw),                                               0,            0];
%H(8,:) = [                                                                             1/Rw,                                            0,                                                      width/(2*Rw),                                               0,            0];

%% ---------------- EKF update ----------------
S = H*P_pred*H' + R;
K = P_pred*H'/(S + 1e-9*eye(size(S)));

x = x_pred + K*(z - z_hat);
Pk = P_pred - K*S*K';

%% ---------------- Output ----------------
xhat = x;
P = Pk;

end

== matlab function generic_truck/TruckMaker/UKF_Articulated_Vehicles ==
  data: z input; u input; xhat output; Q input; R input; Ts input; P output
function [xhat,P] = UKF_TruckTrailer_Robust(z,u,Q,R,Ts)

persistent x Pk

%% INITIALIZATION

if isempty(x)

    % [vx vy r theta Cf Cr Ct]

    x = [15;0.1;0.01;0;5;5;5];

end

if isempty(Pk)

    Pk = diag([1 1 0.1 0.01 5 5 5]);

end


%% PARAMETERS (fill from TruckMaker later)

m  = PARAM.m;
Jz = PARAM.Jz;

mt = PARAM.mt;

lf = PARAM.lf;
lr = PARAM.lr;

lh = PARAM.lh;     % hitch distance
lt = PARAM.lt;     % trailer axle distance

g = 9.82;


%% INPUTS

delta = u(1);
Fx    = u(2);

ay_meas = z(2);


%% EXCITATION CHECK

excitation = abs(ay_meas) > 0.3 && abs(delta) > 0.5*pi/180;


%% UKF PARAMETERS

n = length(x);

W0 = 1 - n/3;
Wi = (1-W0)/(2*n);
gamma = sqrt(n/(1-W0));

Pk = (Pk+Pk')/2 + 1e-9*eye(n);

S = chol(Pk,'lower');


%% SIGMA POINTS

X = zeros(n,2*n+1);
X(:,1) = x;

for i=1:n

    X(:,i+1)   = x + gamma*S(:,i);
    X(:,i+1+n) = x - gamma*S(:,i);

end


%% PROPAGATION

X_pred = zeros(n,2*n+1);

for k=1:2*n+1

vx = X(1,k);
vy = X(2,k);
r  = X(3,k);
theta = X(4,k);

Cf = X(5,k);
Cr = X(6,k);
Ct = X(7,k);


%% SLIP ANGLES

alpha_f = delta - atan2(vy + lf*r , max(vx,0.5));

alpha_r = -atan2(vy - lr*r , max(vx,0.5));

alpha_t = -atan2(vy - (lr+lt)*r + lh*r , max(vx,0.5));


%% NORMAL FORCES

Ffz = PARAM.Ffz;
Frz = PARAM.Frz;

Ftz = PARAM.Ftz;


%% LATERAL FORCES

Fy_f = Cf * alpha_f * Ffz;

Fy_r = Cr * alpha_r * Frz;

Fy_t = Ct * alpha_t * Ftz;


%% VEHICLE DYNAMICS

dvx = Fx/m + vy*r;

dvy = (Fy_f*cos(delta) + Fy_r + Fy_t)/(m+mt) - vx*r;

dr  = (-lf*Fy_f*cos(delta) + lr*Fy_r - lh*Fy_t)/Jz;


%% ARTICULATION

dtheta = r - (vy - (lr+lt)*r)/lh;


%% PROPAGATION

X_pred(:,k) = [

vx + Ts*dvx
vy + Ts*dvy
r  + Ts*dr
theta + Ts*dtheta
Cf
Cr
Ct

];

end


%% MEAN

x_pred = W0*X_pred(:,1);

for k=2:2*n+1

x_pred = x_pred + Wi*X_pred(:,k);

end


%% COVARIANCE

P_pred = Q;

for k=1:2*n+1

w = (k==1)*W0 + (k>1)*Wi;

dx = X_pred(:,k)-x_pred;

P_pred = P_pred + w*(dx*dx');

end


%% MEASUREMENT MODEL

Z = zeros(length(z),2*n+1);

for k=1:2*n+1

vx = X_pred(1,k);
vy = X_pred(2,k);
r  = X_pred(3,k);

ax = Fx/m + vy*r;

ay = -vx*r;

Z(:,k) = [

ax
ay
vx
vy
r

];

end


%% MEASUREMENT MEAN

z_pred = W0*Z(:,1);

for k=2:2*n+1

z_pred = z_pred + Wi*Z(:,k);

end


%% MEASUREMENT COV

S_cov = R;

for k=1:2*n+1

w = (k==1)*W0 + (k>1)*Wi;

dz = Z(:,k)-z_pred;

S_cov = S_cov + w*(dz*dz');

end


%% CROSS COV

Pxz = zeros(n,length(z));

for k=1:2*n+1

w = (k==1)*W0 + (k>1)*Wi;

dx = X_pred(:,k)-x_pred;

dz = Z(:,k)-z_pred;

Pxz = Pxz + w*(dx*dz');

end


%% UPDATE

K = Pxz / S_cov;

x = x_pred + K*(z - z_pred);

Pk = P_pred - K*S_cov*K';


%% ROBUST CONSTRAINTS

x(5) = min(max(x(5),0.01),20);   % Cf

x(6) = min(max(x(6),0.01),20);   % Cr

x(7) = min(max(x(7),0.01),20);   % Ct


%% EXCITATION FREEZE

if ~excitation

x(5:7) = x_pred(5:7);

end


%% ARTICULATION LIMIT

if abs(x(4)) > 20*pi/180

x(7) = x_pred(7);

end


xhat = x;

P = Pk;

end

== matlab function generic_truck/TruckMaker/MATLAB Function ==
  data: u input; y output
function y = fcn(u)

y = u;

== matlab function generic_truck/TruckMaker/Subsystem1/Subsystem/Ackerman Angle/MATLAB Function ==
  data: delta_l input; delta output; delta_r input
function delta = ackerman_angle(delta_l, delta_r)

delta = acot((cot(delta_l) + cot(delta_r))/2);

end

== matlab function generic_truck/TruckMaker/Subsystem1/Subsystem_Noisey Measurements/MATLAB Function ==
  data: gyro_true input; gyro_meas output
function gyro_meas = imu_gyro_noise(gyro_true)

Fs = 1000;   % sample rate

[meas, ~] = GyroNoise(gyro_true', Fs);

gyro_meas = meas';

end

== matlab function generic_truck/TruckMaker/Subsystem1/Subsystem_Noisey Measurements/MATLAB Function1 ==
  data: acc_true input; acc_meas output
function acc_meas = AccelNoiseBlock(acc_true)

Fs = 1000;

truth = acc_true;      % 1×3

[meas,~] = AccelNoise(truth,Fs);

acc_meas = meas;       % 3×1

end

== matlab function generic_truck/TruckMaker/Subsystem1/Subsystem_Noisey Measurements/MATLAB Function2 ==
  data: truth input; vel_meas output
function vel_meas = imu_vel_noise(truth)
    

sigma = 0.05; % m/s^2 (tune later)

vel_meas = truth + sigma * randn(size(truth));


end

== matlab function generic_truck/TruckMaker/Subsystem1/ONE_TRACK_MODEL_TRACTOR_UKF/Working Model with 5 measurements  ==
  data: z input; u input; xhat output; Q input; R input; Ts input; P output; dxdt output; innovation output; K_out output; S_out output; z_pred_out output
function [xhat, P, dxdt, innovation, K_out, S_out, z_pred_out] = UKF_OneTrack_IMU(z, u, Q, R, Ts)

% z = [ax; ay; vx; vy; wz]

%% =========================
%% PERSISTENT VARIABLES
%% =========================
persistent x Pk dxdt_old t

if isempty(x)
    x = [15;0.1;0.1;7.5;7.5];   % [vx vy wz Cf Cr]
end
if isempty(Pk)
    Pk = diag([0.1 0.1 0.1 2 2]);
end
if isempty(dxdt_old)
    dxdt_old = zeros(5,1);
end
if isempty(t)
    t = 0;
end

%% =========================
%% TIME UPDATE
%% =========================
t = t + 0.001;

start_time = 30;
if t < start_time
    xhat = x;
    P = Pk;
    dxdt = dxdt_old;

    innovation = zeros(length(z),1);
    K_out = zeros(length(x), length(z));
    S_out = eye(length(z));
    z_pred_out = zeros(length(z),1);
    return
end

%% =========================
%% VEHICLE PARAMETERS
%% =========================
m  = 6800;
g  = 9.82;
Jz = 12994.917;

p_cog = [3.473;0;0.925];
p_fax = [4.520;0;0.490];
p_rax = [0.950;0;0.490];
p_imu = [3.600;0;1.000];

lf = abs(p_fax(1)-p_cog(1));
lr = abs(p_cog(1)-p_rax(1));
L  = lf + lr;
h  = p_cog(3);

Rfax = p_fax - p_cog; Rfax(3) = -p_cog(3);
Rrax = p_rax - p_cog; Rrax(3) = -p_cog(3);
Rcog = p_imu - p_cog;

%% =========================
%% INPUTS
%% =========================
delta = u(1);
T_rl  = u(2);
T_rr  = u(3);
Rwheel = 0.505;

Fx_vehicle = (T_rl + T_rr)/(Rwheel);

%% =========================
%% UKF PARAMETERS
%% =========================
n = length(x);
W0 = 1 - n/3;
Wi = (1 - W0)/(2*n);
gamma = sqrt(n/(1-W0));

Pk = (Pk+Pk')/2 + 1e-9*eye(n);
S = chol(Pk,'lower');

%% =========================
%% SIGMA POINTS
%% =========================
X = zeros(n,2*n+1);
X(:,1) = x;

for i=1:n
    X(:,i+1)   = x + gamma*S(:,i);
    X(:,i+1+n) = x - gamma*S(:,i);
end

%% =========================
%% PREDICTION
%% =========================
X_pred = zeros(n,2*n+1);
dxdt_model = zeros(5,1);

for k=1:2*n+1

    vx = X(1,k);
    vy = X(2,k);
    wz = X(3,k);
    Cf = X(4,k);
    Cr = X(5,k);

    v_cog = [vx;vy;0];
    omega = [0;0;wz];

    Rotf = [cos(delta) -sin(delta) 0;
            sin(delta)  cos(delta) 0;
            0 0 1];

    vf = Rotf.'*(v_cog + cross(omega,Rfax));
    vr = v_cog + cross(omega,Rrax);

    alpha_f = atan2(vf(2), max(abs(vf(1)),0.1));
    alpha_r = atan2(vr(2), max(abs(vr(1)),0.1));

    ax_est = Fx_vehicle/m + vy*wz;

    Ffz = m*g*lr/L - m*ax_est*h/L;
    Frz = m*g*lf/L + m*ax_est*h/L;

    Fy_f = -Cf * alpha_f * Ffz;
    Fy_r = -Cr * alpha_r * Frz;

    dvx = (Fx_vehicle - Fy_f*sin(delta))/m + vy*wz;
    dvy = (Fy_f*cos(delta) + Fy_r)/m - vx*wz;
    dwz = (lf*Fy_f*cos(delta) - lr*Fy_r)/Jz;

    if k==1
        dxdt_model = [dvx; dvy; dwz; 0; 0];
    end

    X_pred(:,k) = [
        vx + Ts*dvx
        vy + Ts*dvy
        wz + Ts*dwz
        Cf
        Cr
    ];
end

%% =========================
%% MEAN + COV
%% =========================
x_pred = W0*X_pred(:,1);
for k=2:2*n+1
    x_pred = x_pred + Wi*X_pred(:,k);
end

P_pred = zeros(n);
for k=1:2*n+1
    w = (k==1)*W0 + (k>1)*Wi;
    dx = X_pred(:,k)-x_pred;
    P_pred = P_pred + w*(dx*dx');
end
P_pred = P_pred + Q*Ts;

%% =========================
%% MEASUREMENT MODEL
%% =========================
Z = zeros(length(z),2*n+1);

for k=1:2*n+1

    vx = X_pred(1,k);
    vy = X_pred(2,k);
    wz = X_pred(3,k);
    Cf = X_pred(4,k);
    Cr = X_pred(5,k);

    v_cog = [vx;vy;0];
    omega = [0;0;wz];

    Rotf = [cos(delta) -sin(delta) 0;
            sin(delta)  cos(delta) 0;
            0 0 1];

    vf = Rotf.'*(v_cog + cross(omega,Rfax));
    vr = v_cog + cross(omega,Rrax);

    alpha_f = atan2(vf(2), max(abs(vf(1)),0.1));
    alpha_r = atan2(vr(2), max(abs(vr(1)),0.1));

    ax_est = Fx_vehicle/m + vy*wz;

    Ffz = m*g*lr/L - m*ax_est*h/L;
    Frz = m*g*lf/L + m*ax_est*h/L;

    Fy_f = -Cf * alpha_f * Ffz;
    Fy_r = -Cr * alpha_r * Frz;

    dvx = (Fx_vehicle - Fy_f*sin(delta))/m;
    dvy = (Fy_f*cos(delta) + Fy_r)/m;
    dwz = (lf*Fy_f*cos(delta) - lr*Fy_r)/Jz;

    a_cog = [dvx; dvy; 0];
    alpha_vec = [0;0;dwz];

    a_imu = a_cog + cross(omega,cross(omega,Rcog)) + cross(alpha_vec,Rcog);
    v_imu = v_cog + cross(omega,Rcog);

    Z(:,k) = [a_imu(1:2); v_imu(1:2); wz];
end

%% =========================
%% HANDLE NaN MEASUREMENTS
%% =========================
valid_idx = ~isnan(z);

z_used      = z(valid_idx);
z_pred      = W0*Z(:,1);
for k=2:2*n+1
    z_pred = z_pred + Wi*Z(:,k);
end

z_pred_used = z_pred(valid_idx);
Z_used      = Z(valid_idx,:);
R_used      = R(valid_idx, valid_idx);

%% =========================
%% S
%% =========================
S_cov = zeros(length(z_used));
for k=1:2*n+1
    w = (k==1)*W0 + (k>1)*Wi;
    dz = Z_used(:,k)-z_pred_used;
    S_cov = S_cov + w*(dz*dz');
end
S_cov = S_cov + R_used;

%% =========================
%% Pxz
%% =========================
Pxz = zeros(n,length(z_used));
for k=1:2*n+1
    w = (k==1)*W0 + (k>1)*Wi;
    dx = X_pred(:,k)-x_pred;
    dz = Z_used(:,k)-z_pred_used;
    Pxz = Pxz + w*(dx*dz');
end

%% =========================
%% UPDATE
%% =========================
K = Pxz / S_cov;

x = x_pred + K*(z_used - z_pred_used);
Pk = P_pred - K*S_cov*K';
Pk = (Pk+Pk')/2 + 1e-9*eye(n);

%% =========================
%% OUTPUTS
%% =========================
dxdt_old = dxdt_model;

xhat = x;
P = Pk;
dxdt = dxdt_old;

innovation = zeros(length(z),1);
innovation(valid_idx) = z_used - z_pred_used;

K_out = zeros(n,length(z));
K_out(:,valid_idx) = K;

S_out = zeros(length(z));
S_out(valid_idx,valid_idx) = S_cov;

z_pred_out = z_pred;

end

== matlab function generic_truck/TruckMaker/Subsystem1/Subsystem_Noisey Measurements _NAN/MATLAB Function ==
  data: gyro_true input; gyro_meas output
function gyro_meas = imu_gyro_noise(gyro_true)

Fs = 1000;   % sample rate

[meas, ~] = GyroNoise(gyro_true', Fs);

gyro_meas = meas';

end

== matlab function generic_truck/TruckMaker/Subsystem1/Subsystem_Noisey Measurements _NAN/MATLAB Function1 ==
  data: acc_true input; acc_meas output
function acc_meas = AccelNoiseBlock(acc_true)

Fs = 1000;

truth = acc_true;      % 1×3

[meas,~] = AccelNoise(truth,Fs);

acc_meas = meas;       % 3×1

end

== matlab function generic_truck/TruckMaker/Subsystem1/Subsystem_Noisey Measurements _NAN/MATLAB Function2 ==
  data: truth input; vel_meas output
function vel_meas = imu_vel_noise(truth)
    

sigma = 0.05; % m/s^2 (tune later)

vel_meas = truth + sigma * randn(size(truth));


end

== matlab function generic_truck/TruckMaker/Subsystem1/Subsystem_Noisey Measurements _NAN/MATLAB Function3 ==
  data: truth input; vel_meas output
function vel_meas = imu_vel_noise(truth)
    

sigma = 0.05; % m/s^2 (tune later)

vel_meas = truth + sigma * randn(size(truth));


end
